simulink model "mrefrobotarm_modified_previous_y_previous_u_previous_ref_cover"  (R2018b)
settings: Solver=FixedStepAuto  StartTime=0.0  StopTime=20  RelTol=1e-3  AbsTol=1e-6
undefined symbols (not defined in the file or in its folder): cc, options
libraries: neural x396, simulink x1
(part 9 of 15)

== system mrefrobotarm_modified_previous_y_previous_u_previous_ref_cover/cov_no_error/Layer 3/Delays 1 ==
  "p{3}" : Inport  PortDimensions=30
      mask Display: e = 0.06;c1 = [120 230 180]/255;c2 = ([120 230 180]+0)/(256+128);c3 = ([120 230 180]+128)/(256+128);patch([0 1 1 0],[0 0 1 1],c1);patch([0 1 1 1-e 1-e 0+e],[0 0 1 1-e 0+e 0+e],c2);patch([0 0 1 1-e 0+e 0+e],[0 1 1 1-e 1-e 0+e],c3);plot([0 1 1 0 0],[0 0 1 1 0]);
  mux : Mux  Inputs=1
      mask Display: e = 0.06;c1 = [120 150 230]/255;c2 = ([120 150 230]+0)/383;c3 = ([120 150 230]+128)/383;patch([0 1 1 0],[0 0 1 1],c1);patch([0 1 1 1-e 1-e 0+e],[0 0 1 1-e 0+e 0+e],c2);patch([0 0 1 1-e 0+e 0+e],[0 1 1 1-e 1-e 0+e],c3);plot([0 1 1 0 0],[0 0 1 1 0]);disp('Mux')
  "pd{3,2}" : Outport
      mask Display: e = 0.06;c1 = [120 230 180]/255;c2 = ([120 230 180]+0)/(256+128);c3 = ([120 230 180]+128)/(256+128);patch([0 1 1 0],[0 0 1 1],c1);patch([0 1 1 1-e 1-e 0+e],[0 0 1 1-e 0+e 0+e],c2);patch([0 0 1 1-e 0+e 0+e],[0 1 1 1-e 1-e 0+e],c3);plot([0 1 1 0 0],[0 0 1 1 0]);
  wires:
  "p{3}"/1 -> mux/1
  mux/1 -> "pd{3,2}"/1

== system mrefrobotarm_modified_previous_y_previous_u_previous_ref_cover/cov_no_error/Layer 3/LW{3,2} ==
  "ad{3,2}" : Inport  PortDimensions=30
      mask Display: e = 0.06;c1 = [120 230 180]/255;c2 = ([120 230 180]+0)/(256+128);c3 = ([120 230 180]+128)/(256+128);patch([0 1 1 0],[0 0 1 1],c1);patch([0 1 1 1-e 1-e 0+e],[0 0 1 1-e 0+e 0+e],c2);patch([0 0 1 1-e 0+e 0+e],[0 1 1 1-e 1-e 0+e],c3);plot([0 1 1 0 0],[0 0 1 1 0]);
  "IW{3,2}(1,:)'" : Constant  Value=[-0.1379452230534165824149539503196137957274913787841796875;-0.197336135682137092661747601596289314329624176025390625;-0.1841171805882172718416001089281053282320499420166015625;0.06665546447370573890367495550890453159809112548828125;-0.06545064166549481587953351890973863191902637481689453125;0.318094180225835410080748033578856848180294036865234375;-0.27934965619511753498471762213739566504955291748046875;0.0139935365925980027823616325122202397324144840240478515625;-0.455486141451791837209128743779729120433330535888671875;0.3772677800541470727324622203013859689235687255859375;-0.453393383149610251781069791832123883068561553955078125;0.470969447348426439869939486015937291085720062255859375;-0.3286468270716367268136082202545367181301116943359375;0.320584888861692451911267198738642036914825439453125;-0.464539768441674272292374325843411497771739959716796875;-0.25270043137810571654000568742048926651477813720703125;-0.54848573091240038213101115616154856979846954345703125;0.034643075497777321702930208857651450671255588531494140625;0.11104375159022956964793849010675330646336078643798828125;0.265549053558387371243298957779188640415668487548828125;-0.1577902692516034710568106902428553439676761627197265625;-0.422139590908262196666811405521002598106861114501953125;0.055925327579258575505516404291483922861516475677490234375;0.30493478505474758133431123496848158538341522216796875;0.41384271088268775873331151160527952015399932861328125;-0.0273406793315486736084540808633391861803829669952392578125;-0.367773882448511557630155266451765783131122589111328125;-0.27640550052625167953834761647158302366733551025390625;0.29761897331883890860382280152407474815845489501953125;-0.08929812342511929401656090021788259036839008331298828125]
      mask Display: e = 0.06;c1 = [120 150 230]/255;c2 = ([120 150 230]+0)/383;c3 = ([120 150 230]+128)/383;patch([0 1 1 0],[0 0 1 1],c1);patch([0 1 1 1-e 1-e 0+e],[0 0 1 1-e 0+e 0+e],c2);patch([0 0 1 1-e 0+e 0+e],[0 1 1 1-e 1-e 0+e],c3);plot([0 1 1 0 0],[0 0 1 1 0]);disp('weights');
  Mux : Mux  Inputs=1
      mask Display: e = 0.06;c1 = [120 150 230]/255;c2 = ([120 150 230]+0)/383;c3 = ([120 150 230]+128)/383;patch([0 1 1 0],[0 0 1 1],c1);patch([0 1 1 1-e 1-e 0+e],[0 0 1 1-e 0+e 0+e],c2);patch([0 0 1 1-e 0+e 0+e],[0 1 1 1-e 1-e 0+e],c3);plot([0 1 1 0 0],[0 0 1 1 0]);disp('Mux');
  dotprod1 : neural/Weight Functions/dotprod
  "lz{3,2}" : Outport
      mask Display: e = 0.06;c1 = [120 230 180]/255;c2 = ([120 230 180]+0)/(256+128);c3 = ([120 230 180]+128)/(256+128);patch([0 1 1 0],[0 0 1 1],c1);patch([0 1 1 1-e 1-e 0+e],[0 0 1 1-e 0+e 0+e],c2);patch([0 0 1 1-e 0+e 0+e],[0 1 1 1-e 1-e 0+e],c3);plot([0 1 1 0 0],[0 0 1 1 0]);
  wires:
  "IW{3,2}(1,:)'"/1 -> dotprod1/1
  "ad{3,2}"/1 -> dotprod1/2
  dotprod1/1 -> Mux/1
  Mux/1 -> "lz{3,2}"/1

== system mrefrobotarm_modified_previous_y_previous_u_previous_ref_cover/mape/Layer 1/Delays 1 ==
  "p{1}" : Inport  PortDimensions=10
      mask Display: e = 0.06;c1 = [120 230 180]/255;c2 = ([120 230 180]+0)/(256+128);c3 = ([120 230 180]+128)/(256+128);patch([0 1 1 0],[0 0 1 1],c1);patch([0 1 1 1-e 1-e 0+e],[0 0 1 1-e 0+e 0+e],c2);patch([0 0 1 1-e 0+e 0+e],[0 1 1 1-e 1-e 0+e],c3);plot([0 1 1 0 0],[0 0 1 1 0]);
  mux : Mux  Inputs=1
      mask Display: e = 0.06;c1 = [120 150 230]/255;c2 = ([120 150 230]+0)/383;c3 = ([120 150 230]+128)/383;patch([0 1 1 0],[0 0 1 1],c1);patch([0 1 1 1-e 1-e 0+e],[0 0 1 1-e 0+e 0+e],c2);patch([0 0 1 1-e 0+e 0+e],[0 1 1 1-e 1-e 0+e],c3);plot([0 1 1 0 0],[0 0 1 1 0]);disp('Mux')
  "pd{1,1}" : Outport
      mask Display: e = 0.06;c1 = [120 230 180]/255;c2 = ([120 230 180]+0)/(256+128);c3 = ([120 230 180]+128)/(256+128);patch([0 1 1 0],[0 0 1 1],c1);patch([0 1 1 1-e 1-e 0+e],[0 0 1 1-e 0+e 0+e],c2);patch([0 0 1 1-e 0+e 0+e],[0 1 1 1-e 1-e 0+e],c3);plot([0 1 1 0 0],[0 0 1 1 0]);
  wires:
  "p{1}"/1 -> mux/1
  mux/1 -> "pd{1,1}"/1

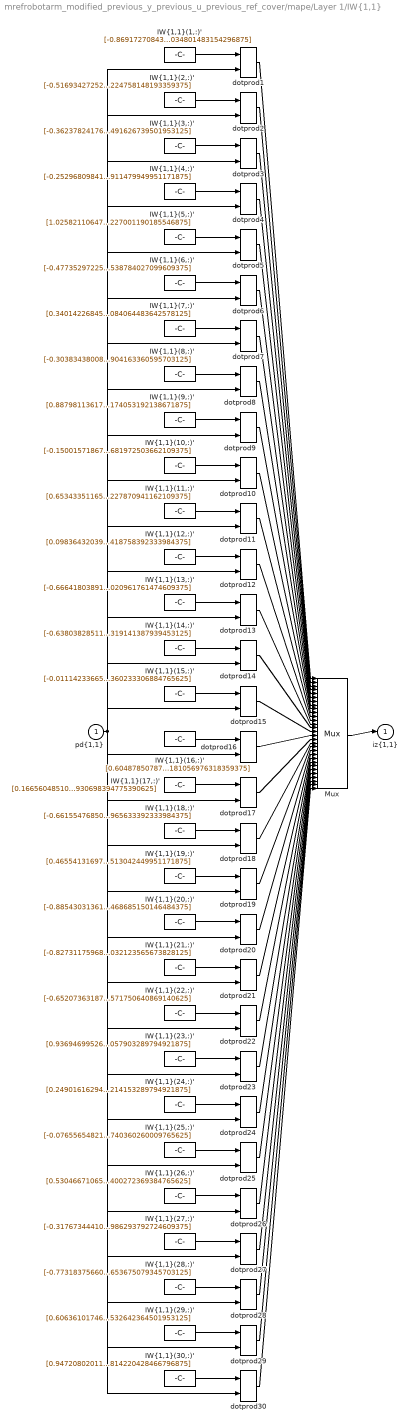
== system mrefrobotarm_modified_previous_y_previous_u_previous_ref_cover/mape/Layer 1/IW{1,1} ==
  "pd{1,1}" : Inport  PortDimensions=10
      mask Display: e = 0.06;c1 = [120 230 180]/255;c2 = ([120 230 180]+0)/(256+128);c3 = ([120 230 180]+128)/(256+128);patch([0 1 1 0],[0 0 1 1],c1);patch([0 1 1 1-e 1-e 0+e],[0 0 1 1-e 0+e 0+e],c2);patch([0 0 1 1-e 0+e 0+e],[0 1 1 1-e 1-e 0+e],c3);plot([0 1 1 0 0],[0 0 1 1 0]);
  "IW{1,1}(1,:)'" : Constant  Value=[-0.86917270843186855699968873523175716400146484375;0.333860251536295227214878877930459566414356231689453125;-0.7652987627475817955513548440649174153804779052734375;-0.209863706009084161063782403289224021136760711669921875;0.976265247910982569834459354751743376255035400390625;0.10643945401961675545354779615081497468054294586181640625;-1.24263877471977313149409383186139166355133056640625;-0.007934239701076629958098607175998040474951267242431640625;0.0706185306788919830989215142835746519267559051513671875;-0.280094379730184417365279614386963658034801483154296875]
      mask Display: e = 0.06;c1 = [120 150 230]/255;c2 = ([120 150 230]+0)/383;c3 = ([120 150 230]+128)/383;patch([0 1 1 0],[0 0 1 1],c1);patch([0 1 1 1-e 1-e 0+e],[0 0 1 1-e 0+e 0+e],c2);patch([0 0 1 1-e 0+e 0+e],[0 1 1 1-e 1-e 0+e],c3);plot([0 1 1 0 0],[0 0 1 1 0]);disp('Weights');
  "IW{1,1}(10,:)'" : Constant  Value=[-0.1500157186735737446792171567722107283771038055419921875;0.378969850924854301243982490632333792746067047119140625;-0.8885808573013165290177539645810611546039581298828125;-1.06526383027227922184465569444000720977783203125;0.002806893424471912888706892630352740525268018245697021484375;0.7194184500055860187472944744513370096683502197265625;-0.1121023282486768579691016611832310445606708526611328125;0.9181583846798064829641816686489619314670562744140625;0.2652202312202562861642718416987918317317962646484375;-0.72833885332476844265414683832204900681972503662109375]
      mask Display: e = 0.06;c1 = [120 150 230]/255;c2 = ([120 150 230]+0)/383;c3 = ([120 150 230]+128)/383;patch([0 1 1 0],[0 0 1 1],c1);patch([0 1 1 1-e 1-e 0+e],[0 0 1 1-e 0+e 0+e],c2);patch([0 0 1 1-e 0+e 0+e],[0 1 1 1-e 1-e 0+e],c3);plot([0 1 1 0 0],[0 0 1 1 0]);disp('Weights');
  "IW{1,1}(11,:)'" : Constant  Value=[0.65343351165336660546500979762640781700611114501953125;-0.318511360012036559563597393207601271569728851318359375;-0.63982827739381342713187450499390251934528350830078125;0.2440570945410153458343671672992059029638767242431640625;0.49755812835218227174749472396797500550746917724609375;1.18749819426796232590959334629587829113006591796875;0.4999897069953933570474191583343781530857086181640625;1.0343322369122749382341908130911178886890411376953125;-0.65342651308895660644537883854354731738567352294921875;-0.76245769669591501038752312524593435227870941162109375]
      mask Display: e = 0.06;c1 = [120 150 230]/255;c2 = ([120 150 230]+0)/383;c3 = ([120 150 230]+128)/383;patch([0 1 1 0],[0 0 1 1],c1);patch([0 1 1 1-e 1-e 0+e],[0 0 1 1-e 0+e 0+e],c2);patch([0 0 1 1-e 0+e 0+e],[0 1 1 1-e 1-e 0+e],c3);plot([0 1 1 0 0],[0 0 1 1 0]);disp('Weights');
  "IW{1,1}(12,:)'" : Constant  Value=[0.09836432039885510680843339059720165096223354339599609375;0.51212284948459629863037889663246460258960723876953125;-0.65129135191145959282721378258429467678070068359375;-0.42588023745715208878692692451295442879199981689453125;-0.99054196117566750690031085468945093452930450439453125;-0.003167554467546782916154146647613742970861494541168212890625;-1.1885297909333498722617150633595883846282958984375;0.447177260773883755717861276934854686260223388671875;0.9631220054162898946970017277635633945465087890625;0.481636324519325087489818315589218400418758392333984375]
      mask Display: e = 0.06;c1 = [120 150 230]/255;c2 = ([120 150 230]+0)/383;c3 = ([120 150 230]+128)/383;patch([0 1 1 0],[0 0 1 1],c1);patch([0 1 1 1-e 1-e 0+e],[0 0 1 1-e 0+e 0+e],c2);patch([0 0 1 1-e 0+e 0+e],[0 1 1 1-e 1-e 0+e],c3);plot([0 1 1 0 0],[0 0 1 1 0]);disp('Weights');
  "IW{1,1}(13,:)'" : Constant  Value=[-0.66641803891031725637361660119495354592800140380859375;0.6494123093341064301142750991857610642910003662109375;-0.43184193032284567959067089759628288447856903076171875;0.08224813599015652620938254813154344446957111358642578125;0.34460417460573500303411265122122131288051605224609375;-0.50998777411279772042718150260043330490589141845703125;0.20825606830708542904773139525786973536014556884765625;-1.3671251686788183921095196637907065451145172119140625;0.361749169071578113854315006392425857484340667724609375;0.8840471254504540521423905374831520020961761474609375]
      mask Display: e = 0.06;c1 = [120 150 230]/255;c2 = ([120 150 230]+0)/383;c3 = ([120 150 230]+128)/383;patch([0 1 1 0],[0 0 1 1],c1);patch([0 1 1 1-e 1-e 0+e],[0 0 1 1-e 0+e 0+e],c2);patch([0 0 1 1-e 0+e 0+e],[0 1 1 1-e 1-e 0+e],c3);plot([0 1 1 0 0],[0 0 1 1 0]);disp('Weights');
  "IW{1,1}(14,:)'" : Constant  Value=[-0.6380382851166503943574070945032872259616851806640625;-0.00570435011875485009635866617827559821307659149169921875;0.316813656488922623655213328675017692148685455322265625;-0.25556427249746038743438703022547997534275054931640625;0.78806282149067896636296381984720937907695770263671875;0.256121186195543193431234385570860467851161956787109375;-0.9691335532975153821411140597774647176265716552734375;-0.78542422352332474932978811921202577650547027587890625;0.91287078704267632378588359642890281975269317626953125;0.65312256330506290868953556127962656319141387939453125]
      mask Display: e = 0.06;c1 = [120 150 230]/255;c2 = ([120 150 230]+0)/383;c3 = ([120 150 230]+128)/383;patch([0 1 1 0],[0 0 1 1],c1);patch([0 1 1 1-e 1-e 0+e],[0 0 1 1-e 0+e 0+e],c2);patch([0 0 1 1-e 0+e 0+e],[0 1 1 1-e 1-e 0+e],c3);plot([0 1 1 0 0],[0 0 1 1 0]);disp('Weights');
  "IW{1,1}(15,:)'" : Constant  Value=[-0.0111423366574186326338757879739205236546695232391357421875;-0.2108438300503387152762257983340532518923282623291015625;1.0248788617387536437064454730716533958911895751953125;1.03304708971095404734796829870902001857757568359375;-0.0750841135508741874815541450516320765018463134765625;1.00817032501042813663616470876149833202362060546875;-0.2014087892260795487064939379706629551947116851806640625;-0.1917620850263474230334992398638860322535037994384765625;0.428022980261531238443950542205129750072956085205078125;0.70117451249500695187322207857505418360233306884765625]
      mask Display: e = 0.06;c1 = [120 150 230]/255;c2 = ([120 150 230]+0)/383;c3 = ([120 150 230]+128)/383;patch([0 1 1 0],[0 0 1 1],c1);patch([0 1 1 1-e 1-e 0+e],[0 0 1 1-e 0+e 0+e],c2);patch([0 0 1 1-e 0+e 0+e],[0 1 1 1-e 1-e 0+e],c3);plot([0 1 1 0 0],[0 0 1 1 0]);disp('Weights');
  "IW{1,1}(16,:)'" : Constant  Value=[0.604878507872788073740366598940454423427581787109375;-0.5946433247025459944978820203687064349651336669921875;-0.7677228915376199669395873570465482771396636962890625;0.283856949116521928289103016140870749950408935546875;0.684678416472543904802705583279021084308624267578125;-1.099841468180588588410273587214760482311248779296875;-0.39134054449506228134936236529028974473476409912109375;0.7138154532712863709065231887507252395153045654296875;-0.04548099428078743178271992064765072427690029144287109375;0.1732650595155303674399505098335794173181056976318359375]
      mask Display: e = 0.06;c1 = [120 150 230]/255;c2 = ([120 150 230]+0)/383;c3 = ([120 150 230]+128)/383;patch([0 1 1 0],[0 0 1 1],c1);patch([0 1 1 1-e 1-e 0+e],[0 0 1 1-e 0+e 0+e],c2);patch([0 0 1 1-e 0+e 0+e],[0 1 1 1-e 1-e 0+e],c3);plot([0 1 1 0 0],[0 0 1 1 0]);disp('Weights');
  "IW{1,1}(17,:)'" : Constant  Value=[0.166560485109207956355703572626225650310516357421875;0.51436311667441569905889764413586817681789398193359375;-0.0272738210767603482531651337694711401127278804779052734375;-0.91126081482300580471900275369989685714244842529296875;0.61851867307643371152181543948245234787464141845703125;0.816639619670167515863568041822873055934906005859375;0.5695765981040470382623652767506428062915802001953125;-0.127726701245082285840481972627458162605762481689453125;-0.46571715194937757242854559081024490296840667724609375;1.1048393233854165718099693549447692930698394775390625]
      mask Display: e = 0.06;c1 = [120 150 230]/255;c2 = ([120 150 230]+0)/383;c3 = ([120 150 230]+128)/383;patch([0 1 1 0],[0 0 1 1],c1);patch([0 1 1 1-e 1-e 0+e],[0 0 1 1-e 0+e 0+e],c2);patch([0 0 1 1-e 0+e 0+e],[0 1 1 1-e 1-e 0+e],c3);plot([0 1 1 0 0],[0 0 1 1 0]);disp('Weights');
  "IW{1,1}(18,:)'" : Constant  Value=[-0.6615547685098766006461801225668750703334808349609375;0.265549820533966973723494220394059084355831146240234375;-0.186044924374246301024271588175906799733638763427734375;-0.9315804733131318737804349439102225005626678466796875;-0.939277771531056515641466830857098102569580078125;-0.603319836425143751768018773873336613178253173828125;0.2268542365193025600600407187812379561364650726318359375;-0.2367942614416354840667366943307570181787014007568359375;-0.76185716659101287984157124810735695064067840576171875;0.65570312248239959185269754016189835965633392333984375]
      mask Display: e = 0.06;c1 = [120 150 230]/255;c2 = ([120 150 230]+0)/383;c3 = ([120 150 230]+128)/383;patch([0 1 1 0],[0 0 1 1],c1);patch([0 1 1 1-e 1-e 0+e],[0 0 1 1-e 0+e 0+e],c2);patch([0 0 1 1-e 0+e 0+e],[0 1 1 1-e 1-e 0+e],c3);plot([0 1 1 0 0],[0 0 1 1 0]);disp('Weights');
  "IW{1,1}(19,:)'" : Constant  Value=[0.46554131697552969537667877375497482717037200927734375;0.042765522848908769926179473941374453715980052947998046875;-0.9190417505712422663322058724588714540004730224609375;-0.5272435508235309153945991056389175355434417724609375;0.939137887083713263081108379992656409740447998046875;-0.08831740047749138400323687392301508225500583648681640625;-0.934752577678931384497218459728173911571502685546875;-1.0752706770670859004468411512789316475391387939453125;-0.316014620826330971947726311555015854537487030029296875;-0.0448947547567741522822615252152900211513042449951171875]
      mask Display: e = 0.06;c1 = [120 150 230]/255;c2 = ([120 150 230]+0)/383;c3 = ([120 150 230]+128)/383;patch([0 1 1 0],[0 0 1 1],c1);patch([0 1 1 1-e 1-e 0+e],[0 0 1 1-e 0+e 0+e],c2);patch([0 0 1 1-e 0+e 0+e],[0 1 1 1-e 1-e 0+e],c3);plot([0 1 1 0 0],[0 0 1 1 0]);disp('Weights');
  "IW{1,1}(2,:)'" : Constant  Value=[-0.51693427252619716938397687044925987720489501953125;0.038223345803574081125386641133445664308965206146240234375;-1.2513153445653937279047340780380181968212127685546875;-0.054874464318876957358295243238899274729192256927490234375;0.274590022853928916735100074220099486410617828369140625;-0.66269570422983725688226286365534178912639617919921875;-1.4604409369190485268319434908335097134113311767578125;-0.70613653008601906524432934020296670496463775634765625;-0.77256806416255774383472498811897821724414825439453125;-0.9015955466411325058828651890507899224758148193359375]
      mask Display: e = 0.06;c1 = [120 150 230]/255;c2 = ([120 150 230]+0)/383;c3 = ([120 150 230]+128)/383;patch([0 1 1 0],[0 0 1 1],c1);patch([0 1 1 1-e 1-e 0+e],[0 0 1 1-e 0+e 0+e],c2);patch([0 0 1 1-e 0+e 0+e],[0 1 1 1-e 1-e 0+e],c3);plot([0 1 1 0 0],[0 0 1 1 0]);disp('Weights');
  "IW{1,1}(20,:)'" : Constant  Value=[-0.8854303136184371592065645018010400235652923583984375;0.70808526149730244281244040394085459411144256591796875;1.0211831026647661957440504920668900012969970703125;1.001161043407467587940118391998112201690673828125;0.45425000119120040320552789125940762460231781005859375;0.1909611499202052142809549195590079762041568756103515625;0.734322514989135921581464572227559983730316162109375;0.305854259693887631232911417100694961845874786376953125;0.55668524266359675767290582371060736477375030517578125;0.392521761573673744205592583966790698468685150146484375]
      mask Display: e = 0.06;c1 = [120 150 230]/255;c2 = ([120 150 230]+0)/383;c3 = ([120 150 230]+128)/383;patch([0 1 1 0],[0 0 1 1],c1);patch([0 1 1 1-e 1-e 0+e],[0 0 1 1-e 0+e 0+e],c2);patch([0 0 1 1-e 0+e 0+e],[0 1 1 1-e 1-e 0+e],c3);plot([0 1 1 0 0],[0 0 1 1 0]);disp('Weights');
  "IW{1,1}(21,:)'" : Constant  Value=[-0.82731175968702597156578804060700349509716033935546875;0.27692008086166541858119671815074980258941650390625;-1.0177676348085586965908078127540647983551025390625;-1.091542090218194260842210496775805950164794921875;0.5333742185100340815750996625865809619426727294921875;-1.0058244351602052546468257787637412548065185546875;-0.444044651398066980707568518482730723917484283447265625;-0.69178193901079954031274610315449535846710205078125;-0.5072143378135576252674354691407643258571624755859375;0.56319370007835900526771411023219116032123565673828125]
      mask Display: e = 0.06;c1 = [120 150 230]/255;c2 = ([120 150 230]+0)/383;c3 = ([120 150 230]+128)/383;patch([0 1 1 0],[0 0 1 1],c1);patch([0 1 1 1-e 1-e 0+e],[0 0 1 1-e 0+e 0+e],c2);patch([0 0 1 1-e 0+e 0+e],[0 1 1 1-e 1-e 0+e],c3);plot([0 1 1 0 0],[0 0 1 1 0]);disp('Weights');
  "IW{1,1}(22,:)'" : Constant  Value=[-0.6520736318759257077459778884076513350009918212890625;-0.18651366163156180011384321915102191269397735595703125;-1.063858327684404248003602333483286201953887939453125;-1.01690941878097351747101129149086773395538330078125;0.1450642281245416442825302283381461165845394134521484375;-1.48961355139560946980736844125203788280487060546875;-0.392413164150247240069546705854008905589580535888671875;0.77740480677343082316355094008031301200389862060546875;0.4476527585276131038227731551160104572772979736328125;0.42889542926241619458238574225106276571750640869140625]
      mask Display: e = 0.06;c1 = [120 150 230]/255;c2 = ([120 150 230]+0)/383;c3 = ([120 150 230]+128)/383;patch([0 1 1 0],[0 0 1 1],c1);patch([0 1 1 1-e 1-e 0+e],[0 0 1 1-e 0+e 0+e],c2);patch([0 0 1 1-e 0+e 0+e],[0 1 1 1-e 1-e 0+e],c3);plot([0 1 1 0 0],[0 0 1 1 0]);disp('Weights');
  "IW{1,1}(23,:)'" : Constant  Value=[0.93694699526127600552882768170093186199665069580078125;-0.65764294407387235974482564415666274726390838623046875;-0.73146447136240422270958561057341285049915313720703125;0.9153130265300302159658940581721253693103790283203125;0.0169856675724000157068349636801940505392849445343017578125;0.5412317499410976839868681054213084280490875244140625;0.7441553618723073526552980183623731136322021484375;-0.147992290543743243436125567313865758478641510009765625;-0.288440262096569421945702060838812030851840972900390625;0.349899850744534723911982609934057109057903289794921875]
      mask Display: e = 0.06;c1 = [120 150 230]/255;c2 = ([120 150 230]+0)/383;c3 = ([120 150 230]+128)/383;patch([0 1 1 0],[0 0 1 1],c1);patch([0 1 1 1-e 1-e 0+e],[0 0 1 1-e 0+e 0+e],c2);patch([0 0 1 1-e 0+e 0+e],[0 1 1 1-e 1-e 0+e],c3);plot([0 1 1 0 0],[0 0 1 1 0]);disp('Weights');
  "IW{1,1}(24,:)'" : Constant  Value=[0.2490161629434594903198529891596990637481212615966796875;-0.7298796994197334075948901954689063131809234619140625;-0.10824562179367229475257516924102674238383769989013671875;0.09140133652043729017844242434875923208892345428466796875;0.647109561580534897728966825525276362895965576171875;1.0401127834781502823346954755834303796291351318359375;0.73517338643845153711708917398937046527862548828125;0.9463932133370251964521457921364344656467437744140625;-0.83892743617914822262804364072508178651332855224609375;0.53949417051280601498319811071269214153289794921875]
      mask Display: e = 0.06;c1 = [120 150 230]/255;c2 = ([120 150 230]+0)/383;c3 = ([120 150 230]+128)/383;patch([0 1 1 0],[0 0 1 1],c1);patch([0 1 1 1-e 1-e 0+e],[0 0 1 1-e 0+e 0+e],c2);patch([0 0 1 1-e 0+e 0+e],[0 1 1 1-e 1-e 0+e],c3);plot([0 1 1 0 0],[0 0 1 1 0]);disp('Weights');
  "IW{1,1}(25,:)'" : Constant  Value=[-0.0765565482169558719771629284878144972026348114013671875;-0.04039471666585343900823801277510938234627246856689453125;-0.5463772797452246532401431977632455527782440185546875;0.675558458816031048854711116291582584381103515625;-0.5760496815664619685293246220680885016918182373046875;-1.01562331359678825748460440081544220447540283203125;-0.107809973611778298074881377033307217061519622802734375;0.943080747799868834846392928739078342914581298828125;-0.7806220998308013303557117978925816714763641357421875;-0.48404875222729393247078633066848851740360260009765625]
      mask Display: e = 0.06;c1 = [120 150 230]/255;c2 = ([120 150 230]+0)/383;c3 = ([120 150 230]+128)/383;patch([0 1 1 0],[0 0 1 1],c1);patch([0 1 1 1-e 1-e 0+e],[0 0 1 1-e 0+e 0+e],c2);patch([0 0 1 1-e 0+e 0+e],[0 1 1 1-e 1-e 0+e],c3);plot([0 1 1 0 0],[0 0 1 1 0]);disp('Weights');
  "IW{1,1}(26,:)'" : Constant  Value=[0.53046671065052819482588120081345550715923309326171875;0.031419921137227392604618358973311842419207096099853515625;-0.442233478797023682460576310404576361179351806640625;0.454501714558769531748794179293327033519744873046875;-0.1371505429258437491757405268799629993736743927001953125;-0.94564246153025599550545621241326443850994110107421875;0.3101428192769046798815679721883498132228851318359375;1.2744040666308913412052561398013494908809661865234375;0.22573753930537121537014400018961168825626373291015625;-0.705368321714067381122958977357484400272369384765625]
      mask Display: e = 0.06;c1 = [120 150 230]/255;c2 = ([120 150 230]+0)/383;c3 = ([120 150 230]+128)/383;patch([0 1 1 0],[0 0 1 1],c1);patch([0 1 1 1-e 1-e 0+e],[0 0 1 1-e 0+e 0+e],c2);patch([0 0 1 1-e 0+e 0+e],[0 1 1 1-e 1-e 0+e],c3);plot([0 1 1 0 0],[0 0 1 1 0]);disp('Weights');
  "IW{1,1}(27,:)'" : Constant  Value=[-0.317673444108008073971660678580519743263721466064453125;-1.1481026843404082971034085858264006674289703369140625;-0.797589850506532638263479384477250277996063232421875;-0.77800096016235276152883670874871313571929931640625;0.37979337230280940662652255923603661358356475830078125;-0.95217759395398349209216348754125647246837615966796875;-0.769641582911539945399681528215296566486358642578125;-0.37050739846647207098584431150811724364757537841796875;0.446306369913247513725451653954223729670047760009765625;0.77990666245966655534260780768818221986293792724609375]
      mask Display: e = 0.06;c1 = [120 150 230]/255;c2 = ([120 150 230]+0)/383;c3 = ([120 150 230]+128)/383;patch([0 1 1 0],[0 0 1 1],c1);patch([0 1 1 1-e 1-e 0+e],[0 0 1 1-e 0+e 0+e],c2);patch([0 0 1 1-e 0+e 0+e],[0 1 1 1-e 1-e 0+e],c3);plot([0 1 1 0 0],[0 0 1 1 0]);disp('Weights');
  "IW{1,1}(28,:)'" : Constant  Value=[-0.77318375660010130179244924875092692673206329345703125;0.2435390007385561383923544553908868692815303802490234375;0.98530964647025143232639265988836996257305145263671875;0.71632615969698620883576722917496226727962493896484375;0.76099926840397402738602750105201266705989837646484375;-0.53978676857327345661730078063555993139743804931640625;0.2472085844721277625435362779171555303037166595458984375;1.0037419496869304236241760008851997554302215576171875;0.25527208823712854712795206069131381809711456298828125;-0.5379047395273570675300334187340922653675079345703125]
      mask Display: e = 0.06;c1 = [120 150 230]/255;c2 = ([120 150 230]+0)/383;c3 = ([120 150 230]+128)/383;patch([0 1 1 0],[0 0 1 1],c1);patch([0 1 1 1-e 1-e 0+e],[0 0 1 1-e 0+e 0+e],c2);patch([0 0 1 1-e 0+e 0+e],[0 1 1 1-e 1-e 0+e],c3);plot([0 1 1 0 0],[0 0 1 1 0]);disp('Weights');
  "IW{1,1}(29,:)'" : Constant  Value=[0.606361017460992801630936810397543013095855712890625;-0.5372362456303261257772874159854836761951446533203125;0.8026730113580475833856553435907699167728424072265625;-0.270047393454473871887699942817562259733676910400390625;-0.8583397719395209346515684956102631986141204833984375;-0.760775487120716409350507092312909662723541259765625;0.7934160687685019031079036722076125442981719970703125;0.726215606769777810569621578906662762165069580078125;-0.203810811400221225664353141837636940181255340576171875;-0.0279812009177607297349954507126312819309532642364501953125]
      mask Display: e = 0.06;c1 = [120 150 230]/255;c2 = ([120 150 230]+0)/383;c3 = ([120 150 230]+128)/383;patch([0 1 1 0],[0 0 1 1],c1);patch([0 1 1 1-e 1-e 0+e],[0 0 1 1-e 0+e 0+e],c2);patch([0 0 1 1-e 0+e 0+e],[0 1 1 1-e 1-e 0+e],c3);plot([0 1 1 0 0],[0 0 1 1 0]);disp('Weights');
  "IW{1,1}(3,:)'" : Constant  Value=[-0.36237824176308708334914854276576079428195953369140625;-0.6698046119466767311934063400258310139179229736328125;0.608390534767694557416461975662969052791595458984375;-0.7613218350577446447147167418734170496463775634765625;-0.5950203823605180186717689139186404645442962646484375;0.52870201131995020471521229410427622497081756591796875;0.8288893831545907087132718515931628644466400146484375;-0.109983057881297252578178813564591109752655029296875;-0.478212409223443268846409637262695468962192535400390625;-0.8004436614077665712585485380259342491626739501953125]
      mask Display: e = 0.06;c1 = [120 150 230]/255;c2 = ([120 150 230]+0)/383;c3 = ([120 150 230]+128)/383;patch([0 1 1 0],[0 0 1 1],c1);patch([0 1 1 1-e 1-e 0+e],[0 0 1 1-e 0+e 0+e],c2);patch([0 0 1 1-e 0+e 0+e],[0 1 1 1-e 1-e 0+e],c3);plot([0 1 1 0 0],[0 0 1 1 0]);disp('Weights');
  "IW{1,1}(30,:)'" : Constant  Value=[0.94720802011927152097570115074631758034229278564453125;-0.016302704298563119866827264559105969965457916259765625;0.65280419192514316240050220585544593632221221923828125;0.74773890630079187236134430349920876324176788330078125;-0.2487040207870039598692102345012244768440723419189453125;0.96954466205885569962674708222039043903350830078125;0.28518913397178125013198268788983114063739776611328125;-0.5025239053422823065631064309854991734027862548828125;0.779920137708228988770997602841816842555999755859375;-0.539334669681505118887798744253814220428466796875]
      mask Display: e = 0.06;c1 = [120 150 230]/255;c2 = ([120 150 230]+0)/383;c3 = ([120 150 230]+128)/383;patch([0 1 1 0],[0 0 1 1],c1);patch([0 1 1 1-e 1-e 0+e],[0 0 1 1-e 0+e 0+e],c2);patch([0 0 1 1-e 0+e 0+e],[0 1 1 1-e 1-e 0+e],c3);plot([0 1 1 0 0],[0 0 1 1 0]);disp('Weights');
  "IW{1,1}(4,:)'" : Constant  Value=[-0.2529680984142268496128735932870768010616302490234375;0.297710356894141325856395496884942986071109771728515625;0.007280784522140413585200580115497359656728804111480712890625;-0.67077452173686513692274502318468876183032989501953125;0.362267577310952493263584983651526272296905517578125;-1.196968588376917441706837053061462938785552978515625;-0.88745158320561501330558940026094205677509307861328125;-0.77412164849487774542780016417964361608028411865234375;-0.90583798862696174314379504721728153526782989501953125;0.7974738244943793130659059897880069911479949951171875]
      mask Display: e = 0.06;c1 = [120 150 230]/255;c2 = ([120 150 230]+0)/383;c3 = ([120 150 230]+128)/383;patch([0 1 1 0],[0 0 1 1],c1);patch([0 1 1 1-e 1-e 0+e],[0 0 1 1-e 0+e 0+e],c2);patch([0 0 1 1-e 0+e 0+e],[0 1 1 1-e 1-e 0+e],c3);plot([0 1 1 0 0],[0 0 1 1 0]);disp('Weights');
  "IW{1,1}(5,:)'" : Constant  Value=[1.025821106471888288780291986768133938312530517578125;0.1806704307719206592519611831448855809867382049560546875;0.51787573159602329209150184397003613412380218505859375;-0.160972688736257196762124976885388605296611785888671875;-0.04423598861788689828866694142561755143105983734130859375;0.9825514988779768810189807481947354972362518310546875;0.121424311016322061806960164176416583359241485595703125;1.1096047223703198181254947485285811126232147216796875;-0.82412555676097409840252794310799799859523773193359375;0.70930791531166004215691600620630197227001190185546875]
      mask Display: e = 0.06;c1 = [120 150 230]/255;c2 = ([120 150 230]+0)/383;c3 = ([120 150 230]+128)/383;patch([0 1 1 0],[0 0 1 1],c1);patch([0 1 1 1-e 1-e 0+e],[0 0 1 1-e 0+e 0+e],c2);patch([0 0 1 1-e 0+e 0+e],[0 1 1 1-e 1-e 0+e],c3);plot([0 1 1 0 0],[0 0 1 1 0]);disp('Weights');
  "IW{1,1}(6,:)'" : Constant  Value=[-0.477352972254387608597170356006245128810405731201171875;0.266125937652828825630280107361613772809505462646484375;0.45358373296830978294025271679856814444065093994140625;0.7369893069153243825297749935998581349849700927734375;1.1004652600738229484278463132795877754688262939453125;0.65973355375366382613577798110782168805599212646484375;0.80461403048179425123720420742756687104701995849609375;0.5852541899593319829619986194302327930927276611328125;-0.70473714287965083524767351264017634093761444091796875;-1.433412834560731763389185289270244538784027099609375]
      mask Display: e = 0.06;c1 = [120 150 230]/255;c2 = ([120 150 230]+0)/383;c3 = ([120 150 230]+128)/383;patch([0 1 1 0],[0 0 1 1],c1);patch([0 1 1 1-e 1-e 0+e],[0 0 1 1-e 0+e 0+e],c2);patch([0 0 1 1-e 0+e 0+e],[0 1 1 1-e 1-e 0+e],c3);plot([0 1 1 0 0],[0 0 1 1 0]);disp('Weights');
  "IW{1,1}(7,:)'" : Constant  Value=[0.340142268450252915901188544012256897985935211181640625;-0.69589846688402168251030843748594634234905242919921875;-0.6415031322007289649178574109100736677646636962890625;-0.10968082827398893674963886724071926437318325042724609375;-0.77300987038361135272879209878738038241863250732421875;-0.0249272144006855191078475542099113226868212223052978515625;-0.8878367260761559354165228796773590147495269775390625;-0.5784595595146893032278967439197003841400146484375;-0.64828917433955413063273454099544323980808258056640625;-0.67849730996397206173043059607152827084064483642578125]
      mask Display: e = 0.06;c1 = [120 150 230]/255;c2 = ([120 150 230]+0)/383;c3 = ([120 150 230]+128)/383;patch([0 1 1 0],[0 0 1 1],c1);patch([0 1 1 1-e 1-e 0+e],[0 0 1 1-e 0+e 0+e],c2);patch([0 0 1 1-e 0+e 0+e],[0 1 1 1-e 1-e 0+e],c3);plot([0 1 1 0 0],[0 0 1 1 0]);disp('Weights');
  "IW{1,1}(8,:)'" : Constant  Value=[-0.303834380083024047092266073377686552703380584716796875;-0.95241555079364637048655595208401791751384735107421875;0.85746501946415631945086488485685549676418304443359375;0.13583723610552400629103431128896772861480712890625;1.101399410825187441531625154311768710613250732421875;-0.269874602506473160179467640773509629070758819580078125;-0.76381610333243921129309228490456007421016693115234375;0.1679532157508613343654957361650303937494754791259765625;0.1494574362098292918954456354185822419822216033935546875;0.330561366715623361489662102030706591904163360595703125]
      mask Display: e = 0.06;c1 = [120 150 230]/255;c2 = ([120 150 230]+0)/383;c3 = ([120 150 230]+128)/383;patch([0 1 1 0],[0 0 1 1],c1);patch([0 1 1 1-e 1-e 0+e],[0 0 1 1-e 0+e 0+e],c2);patch([0 0 1 1-e 0+e 0+e],[0 1 1 1-e 1-e 0+e],c3);plot([0 1 1 0 0],[0 0 1 1 0]);disp('Weights');
  "IW{1,1}(9,:)'" : Constant  Value=[0.88798113617824181442728104229900054633617401123046875;0.11232248717519406622233901771323871798813343048095703125;1.159371330064498550882490235380828380584716796875;0.126953553855701339880823752537253312766551971435546875;-0.498658128605751371775767211147467605769634246826171875;1.401446477623986108795861582621000707149505615234375;0.76064067156129000490949465529411099851131439208984375;0.176057995679501588792703614672063849866390228271484375;-0.427022019156375443049711293497239239513874053955078125;0.89999126308744592517285809663007967174053192138671875]
      mask Display: e = 0.06;c1 = [120 150 230]/255;c2 = ([120 150 230]+0)/383;c3 = ([120 150 230]+128)/383;patch([0 1 1 0],[0 0 1 1],c1);patch([0 1 1 1-e 1-e 0+e],[0 0 1 1-e 0+e 0+e],c2);patch([0 0 1 1-e 0+e 0+e],[0 1 1 1-e 1-e 0+e],c3);plot([0 1 1 0 0],[0 0 1 1 0]);disp('Weights');
  Mux : Mux  Inputs=30
      mask Display: e = 0.06;c1 = [120 150 230]/255;c2 = ([120 150 230]+0)/383;c3 = ([120 150 230]+128)/383;patch([0 1 1 0],[0 0 1 1],c1);patch([0 1 1 1-e 1-e 0+e],[0 0 1 1-e 0+e 0+e],c2);patch([0 0 1 1-e 0+e 0+e],[0 1 1 1-e 1-e 0+e],c3);plot([0 1 1 0 0],[0 0 1 1 0]);disp('Mux');
  dotprod{1..30} (30 alike) : neural/Weight Functions/dotprod
  "iz{1,1}" : Outport
      mask Display: e = 0.06;c1 = [120 230 180]/255;c2 = ([120 230 180]+0)/(256+128);c3 = ([120 230 180]+128)/(256+128);patch([0 1 1 0],[0 0 1 1],c1);patch([0 1 1 1-e 1-e 0+e],[0 0 1 1-e 0+e 0+e],c2);patch([0 0 1 1-e 0+e 0+e],[0 1 1 1-e 1-e 0+e],c3);plot([0 1 1 0 0],[0 0 1 1 0]);
  wires:
  "IW{1,1}(1,:)'"/1 -> dotprod1/1
  "pd{1,1}"/1 -> dotprod1/2, dotprod2/2, dotprod3/2, dotprod4/2, dotprod5/2, dotprod6/2, dotprod7/2, dotprod8/2, dotprod9/2, dotprod10/2, dotprod11/2, dotprod12/2, dotprod13/2, dotprod14/2, dotprod15/2, dotprod16/2, dotprod17/2, dotprod18/2, dotprod19/2, dotprod20/2, dotprod21/2, dotprod22/2, dotprod23/2, dotprod24/2, dotprod25/2, dotprod26/2, dotprod27/2, dotprod28/2, dotprod29/2, dotprod30/2
  dotprod1/1 -> Mux/1
  "IW{1,1}(2,:)'"/1 -> dotprod2/1
  dotprod2/1 -> Mux/2
  "IW{1,1}(3,:)'"/1 -> dotprod3/1
  dotprod3/1 -> Mux/3
  "IW{1,1}(4,:)'"/1 -> dotprod4/1
  dotprod4/1 -> Mux/4
  "IW{1,1}(5,:)'"/1 -> dotprod5/1
  dotprod5/1 -> Mux/5
  "IW{1,1}(6,:)'"/1 -> dotprod6/1
  dotprod6/1 -> Mux/6
  "IW{1,1}(7,:)'"/1 -> dotprod7/1
  dotprod7/1 -> Mux/7
  "IW{1,1}(8,:)'"/1 -> dotprod8/1
  dotprod8/1 -> Mux/8
  "IW{1,1}(9,:)'"/1 -> dotprod9/1
  dotprod9/1 -> Mux/9
  "IW{1,1}(10,:)'"/1 -> dotprod10/1
  dotprod10/1 -> Mux/10
  "IW{1,1}(11,:)'"/1 -> dotprod11/1
  dotprod11/1 -> Mux/11
  "IW{1,1}(12,:)'"/1 -> dotprod12/1
  dotprod12/1 -> Mux/12
  "IW{1,1}(13,:)'"/1 -> dotprod13/1
  dotprod13/1 -> Mux/13
  "IW{1,1}(14,:)'"/1 -> dotprod14/1
  dotprod14/1 -> Mux/14
  "IW{1,1}(15,:)'"/1 -> dotprod15/1
  dotprod15/1 -> Mux/15
  "IW{1,1}(16,:)'"/1 -> dotprod16/1
  dotprod16/1 -> Mux/16
  "IW{1,1}(17,:)'"/1 -> dotprod17/1
  dotprod17/1 -> Mux/17
  "IW{1,1}(18,:)'"/1 -> dotprod18/1
  dotprod18/1 -> Mux/18
  "IW{1,1}(19,:)'"/1 -> dotprod19/1
  dotprod19/1 -> Mux/19
  "IW{1,1}(20,:)'"/1 -> dotprod20/1
  dotprod20/1 -> Mux/20
  "IW{1,1}(21,:)'"/1 -> dotprod21/1
  dotprod21/1 -> Mux/21
  "IW{1,1}(22,:)'"/1 -> dotprod22/1
  dotprod22/1 -> Mux/22
  "IW{1,1}(23,:)'"/1 -> dotprod23/1
  dotprod23/1 -> Mux/23
  "IW{1,1}(24,:)'"/1 -> dotprod24/1
  dotprod24/1 -> Mux/24
  "IW{1,1}(25,:)'"/1 -> dotprod25/1
  dotprod25/1 -> Mux/25
  "IW{1,1}(26,:)'"/1 -> dotprod26/1
  dotprod26/1 -> Mux/26
  "IW{1,1}(27,:)'"/1 -> dotprod27/1
  dotprod27/1 -> Mux/27
  "IW{1,1}(28,:)'"/1 -> dotprod28/1
  dotprod28/1 -> Mux/28
  "IW{1,1}(29,:)'"/1 -> dotprod29/1
  dotprod29/1 -> Mux/29
  "IW{1,1}(30,:)'"/1 -> dotprod30/1
  dotprod30/1 -> Mux/30
  Mux/1 -> "iz{1,1}"/1

== system mrefrobotarm_modified_previous_y_previous_u_previous_ref_cover/mape/Layer 2/Delays 1 ==
  "p{2}" : Inport  PortDimensions=30
      mask Display: e = 0.06;c1 = [120 230 180]/255;c2 = ([120 230 180]+0)/(256+128);c3 = ([120 230 180]+128)/(256+128);patch([0 1 1 0],[0 0 1 1],c1);patch([0 1 1 1-e 1-e 0+e],[0 0 1 1-e 0+e 0+e],c2);patch([0 0 1 1-e 0+e 0+e],[0 1 1 1-e 1-e 0+e],c3);plot([0 1 1 0 0],[0 0 1 1 0]);
  mux : Mux  Inputs=1
      mask Display: e = 0.06;c1 = [120 150 230]/255;c2 = ([120 150 230]+0)/383;c3 = ([120 150 230]+128)/383;patch([0 1 1 0],[0 0 1 1],c1);patch([0 1 1 1-e 1-e 0+e],[0 0 1 1-e 0+e 0+e],c2);patch([0 0 1 1-e 0+e 0+e],[0 1 1 1-e 1-e 0+e],c3);plot([0 1 1 0 0],[0 0 1 1 0]);disp('Mux')
  "pd{2,1}" : Outport
      mask Display: e = 0.06;c1 = [120 230 180]/255;c2 = ([120 230 180]+0)/(256+128);c3 = ([120 230 180]+128)/(256+128);patch([0 1 1 0],[0 0 1 1],c1);patch([0 1 1 1-e 1-e 0+e],[0 0 1 1-e 0+e 0+e],c2);patch([0 0 1 1-e 0+e 0+e],[0 1 1 1-e 1-e 0+e],c3);plot([0 1 1 0 0],[0 0 1 1 0]);
  wires:
  "p{2}"/1 -> mux/1
  mux/1 -> "pd{2,1}"/1
